simulink model "CL"  (R2017a)
settings: Solver=VariableStepAuto  StartTime=0.0  StopTime=10.0  RelTol=1e-3
values from neighbouring files (symbols this model uses):
  CDLIM = current_limit    [System.m]
  delay_denominator = [-2/(tau_cd)]    [System.m]
  delay_numerator = [2/(tau_cd)]    [System.m]
  DroneMomentArm = MomentArm*milli    [System.m]
  ELEC0_DEN = [M0(TermL),M0(TermR)]    [System.m]
  ELEC0_NUM = [1]    [System.m]
  ELEC1_DEN = [M1(TermL),M1(TermR)]    [System.m]
  ELEC1_NUM = [1]    [System.m]
  linearizedThrustSlope = 2*fittedmodel.p1*(RadSec_SS) + fittedmodel.p2    [Linearization.m]    (also in System.m = 2*lift_coef*RadSec_SS)
  M0 = [ ... (first row only)    [MotorSpecs.m]
  M1 = M0    [System.m]
  MECH0_DEN = [M0(RotJ)+PropellerJ,M0_dyn_fric+linearizedFrictionCoef]    [System.m]
  MECH0_NUM = [1]    [System.m]
  MECH1_DEN = [M1(RotJ)+PropellerJ,M1_dyn_fric+linearizedFrictionCoef]    [System.m]
  MECH1_NUM = [1]    [System.m]
  RadSec_SS = 14000*RadPSecPerRPM    [Linearization.m]    (also in System.m = RPM*RadPSecPerRPM)
  SpdK = 12    [Constants.m]
  Thrust_SS = 1.9794    [System.m]
  TorqueK = 11    [Constants.m]
libraries: simulink x1
settings Model: Creator=Matthew  LastModifiedBy=Matthew

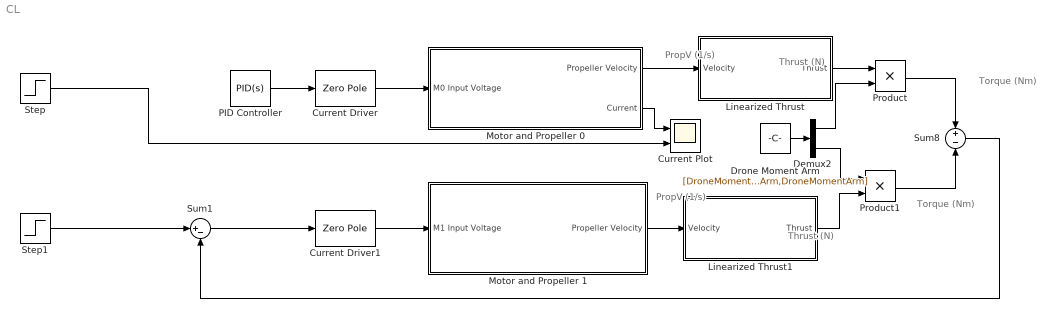
== system CL ==
  note: Thrust (N)
  note: Torque (Nm)
  note: Torque (Nm)
  note: PropV (1/s)
  note: Thrust (N)
  note: PropV (1/s)
  Current Driver : ZeroPole  Zeros=delay_numerator  Poles=delay_denominator  Gain=[-1]
  Current Driver1 : ZeroPole  Zeros=delay_numerator  Poles=delay_denominator  Gain=[-1]
  Current Plot : Scope  NumInputPorts=2
  Demux2 : Demux  Outputs=2
  Drone Moment Arm : Constant  Value=[DroneMomentArm,DroneMomentArm]
  Linearized Thrust : Subsystem
  Linearized Thrust1 : Subsystem
  Motor and Propeller 0 : Subsystem
  Motor and Propeller 1 : Subsystem
  PID Controller : simulink/Continuous/PID Controller  Controller=PID  TimeDomain=Continuous-time  SampleTime=-1  IntegratorMethod=Forward Euler  FilterMethod=Forward Euler  Form=Parallel  UseFilter=on  ControllerParametersSource=internal  P=1  I=1  D=0  N=100  InitialConditionSource=internal  InitialConditionForIntegrator=0  InitialConditionForFilter=0  ExternalReset=none  LimitOutput=off  UpperSaturationLimit=inf  LowerSaturationLimit=-inf  LinearizeAsGain=on  AntiWindupMode=none  Kb=1  TrackingMode=off  Kt=1  PParamMin=[]  PParamMax=[]  IParamMin=[]  IParamMax=[]  DParamMin=[]  DParamMax=[]  NParamMin=[]  NParamMax=[]  KbParamMin=[]  KbParamMax=[]  KtParamMin=[]  KtParamMax=[]  POutMin=[]  POutMax=[]  IOutMin=[]  IOutMax=[]  DOutMin=[]  DOutMax=[]  NOutMin=[]  NOutMax=[]  KbOutMin=[]  KbOutMax=[]  KtOutMin=[]  KtOutMax=[]  IntegratorOutMin=[]  IntegratorOutMax=[]  FilterOutMin=[]  FilterOutMax=[]  SumOutMin=[]  SumOutMax=[]  SumI1OutMin=[]  SumI1OutMax=[]  SumI2OutMin=[]  SumI2OutMax=[]  SumI3OutMin=[]  SumI3OutMax=[]  SumDOutMin=[]  SumDOutMax=[]  SaturationOutMin=[]  SaturationOutMax=[]  IntegratorContinuousStateAttributes=''  IntegratorStateMustResolveToSignalObject=off  IntegratorRTWStateStorageClass=Auto  FilterContinuousStateAttributes=''  FilterStateMustResolveToSignalObject=off  FilterRTWStateStorageClass=Auto  DifferentiatorICPrevScaledInput=0  DifferentiatorOutMin=[]  DifferentiatorOutMax=[]  InitialConditionSetting=State (most efficient)
  Product : Product
  Product1 : Product
  Step : Step  Time=5  After=2  SampleTime=0
  Step1 : Step  Time=5  After=0  SampleTime=0
  Sum1 : Sum  Inputs=|+-
  Sum8 : Sum  Inputs=+|-
  wires:
  Drone Moment Arm/1 -> Demux2/1
  Current Driver1/1 -> Motor and Propeller 1/1(M1 Input Voltage)
  Motor and Propeller 1/1(Propeller Velocity) -> Linearized Thrust1/1(Velocity)
  Linearized Thrust1/1(Thrust) -> Product1/2
  Current Driver/1 -> Motor and Propeller 0/1(M0 Input Voltage)
  Motor and Propeller 0/2(Current) -> Current Plot/1
  Sum8/1 -> Sum1/2
  Demux2/1 -> Product/2
  Linearized Thrust/1(Thrust) -> Product/1
  Product1/1 -> Sum8/2
  Demux2/2 -> Product1/1
  Product/1 -> Sum8/1
  Motor and Propeller 0/1(Propeller Velocity) -> Linearized Thrust/1(Velocity)
  Step1/1 -> Sum1/1
  Sum1/1 -> Current Driver1/1
  Step/1 -> Current Plot/2
  PID Controller/1 -> Current Driver/1

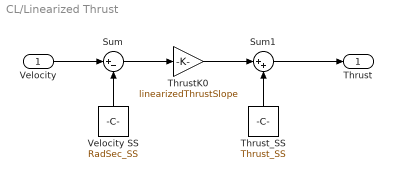
== system CL/Linearized Thrust ==
  Velocity : Inport
  Sum : Sum  Inputs=|+-
  Sum1 : Sum  Inputs=|++
  "ThrustK0 " : Gain  Gain=linearizedThrustSlope
  Thrust_SS : Constant  Value=Thrust_SS
  Velocity SS : Constant  Value=RadSec_SS
  Thrust : Outport
  wires:
  "ThrustK0 "/1 -> Sum1/1
  Sum/1 -> "ThrustK0 "/1
  Sum1/1 -> Thrust/1
  Velocity/1 -> Sum/1
  Velocity SS/1 -> Sum/2
  Thrust_SS/1 -> Sum1/2

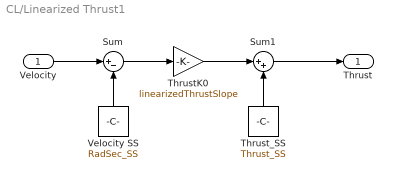
== system CL/Linearized Thrust1 ==
  Velocity : Inport
  Sum : Sum  Inputs=|+-
  Sum1 : Sum  Inputs=|++
  "ThrustK0 " : Gain  Gain=linearizedThrustSlope
  Thrust_SS : Constant  Value=Thrust_SS
  Velocity SS : Constant  Value=RadSec_SS
  Thrust : Outport
  wires:
  "ThrustK0 "/1 -> Sum1/1
  Sum/1 -> "ThrustK0 "/1
  Sum1/1 -> Thrust/1
  Velocity/1 -> Sum/1
  Velocity SS/1 -> Sum/2
  Thrust_SS/1 -> Sum1/2

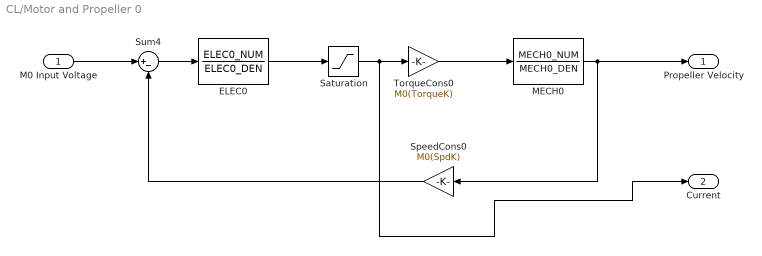
== system CL/Motor and Propeller 0 ==
  M0 Input Voltage : Inport
  ELEC0 : TransferFcn  Numerator=ELEC0_NUM  Denominator=ELEC0_DEN
  MECH0 : TransferFcn  Numerator=MECH0_NUM  Denominator=MECH0_DEN
  Saturation : Saturate  UpperLimit=CDLIM  LowerLimit=0
  SpeedCons0 : Gain  Gain=M0(SpdK)
  Sum4 : Sum  Inputs=|+-
  TorqueCons0 : Gain  Gain=M0(TorqueK)
  Propeller Velocity : Outport
  Current : Outport  Port=2
  wires:
  M0 Input Voltage/1 -> Sum4/1
  Sum4/1 -> ELEC0/1
  TorqueCons0/1 -> MECH0/1
  SpeedCons0/1 -> Sum4/2
  MECH0/1 -> Propeller Velocity/1, SpeedCons0/1
  ELEC0/1 -> Saturation/1
  Saturation/1 -> Current/1, TorqueCons0/1

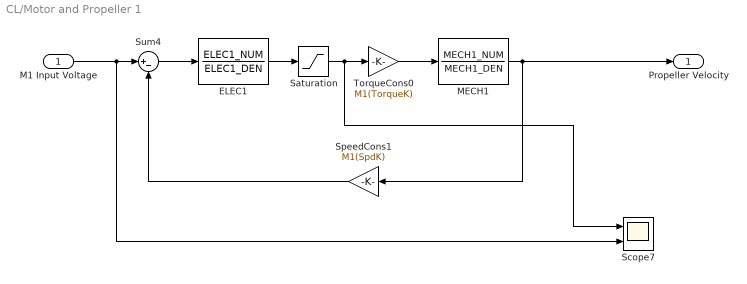
== system CL/Motor and Propeller 1 ==
  M1 Input Voltage : Inport
  ELEC1 : TransferFcn  Numerator=ELEC1_NUM  Denominator=ELEC1_DEN
  MECH1 : TransferFcn  Numerator=MECH1_NUM  Denominator=MECH1_DEN
  Saturation : Saturate  UpperLimit=CDLIM  LowerLimit=0
  Scope7 : Scope  NumInputPorts=2
  SpeedCons1 : Gain  Gain=M1(SpdK)
  Sum4 : Sum  Inputs=|+-
  TorqueCons0 : Gain  Gain=M1(TorqueK)
  Propeller Velocity : Outport
  wires:
  M1 Input Voltage/1 -> Scope7/2, Sum4/1
  Sum4/1 -> ELEC1/1
  TorqueCons0/1 -> MECH1/1
  SpeedCons1/1 -> Sum4/2
  MECH1/1 -> Propeller Velocity/1, SpeedCons1/1
  ELEC1/1 -> Saturation/1
  Saturation/1 -> Scope7/1, TorqueCons0/1
